simulink model "clik_inverse"  (Simulink 10.2)
settings: Solver=ode1  StartTime=0.0  StopTime=4  FixedStep=0.001  RelTol=1e-3
undefined symbols (not defined in the file or in its folder): DiscIntNeverNeededParam, q0, Tc
settings Model: Creator=Xp  LastModifiedBy=Megha
settings DataIOCC: LimitDataPoints=on
settings OptimizationCC: ExpressionDepthLimit=2147483647  InitFltsAndDblsToZero=on
settings DebuggingCC: SaveWithParameterizedLinksMsg=none  SolverPrmCheckMsg=warning  MultiTaskDSMMsg=warning  MultiTaskCondExecSysMsg=none  StateNameClashWarn=warning
settings SFSimCC: SimUseLocalCustomCode=on
settings RTWCC: RTWUseLocalCustomCode=on
settings ConfigComp: CovExternalEMLEnable=on

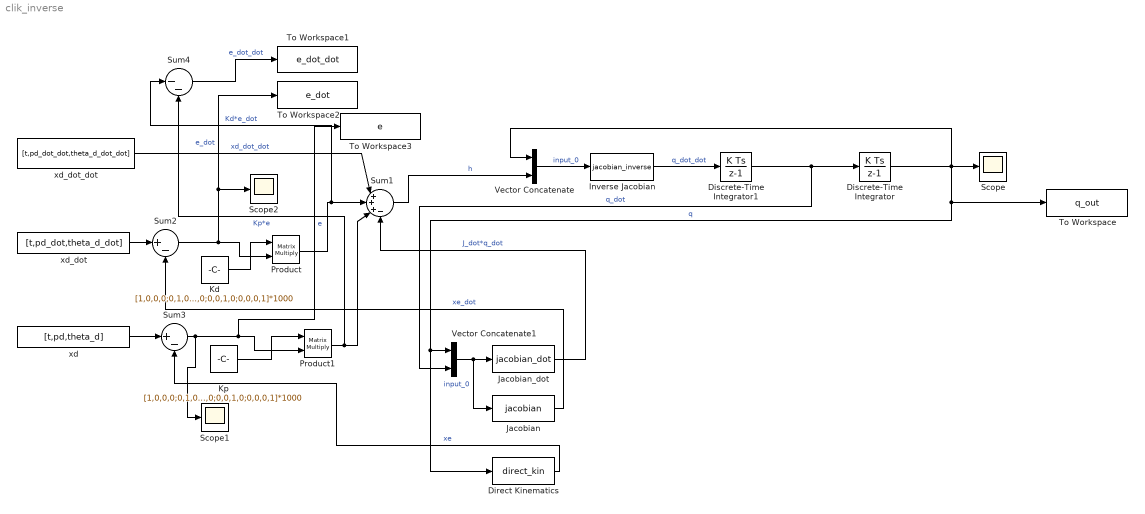
== system clik_inverse ==
  Direct Kinematics : MATLABFcn  MATLABFcn=direct_kin  Output1D=off
  Discrete-Time Integrator : DiscreteIntegrator  InitialCondition=q0  SampleTime=Tc  ICPrevOutput=DiscIntNeverNeededParam  ICPrevScaledInput=DiscIntNeverNeededParam
  Discrete-Time Integrator1 : DiscreteIntegrator  InitialCondition=[0;0;0;0]  SampleTime=Tc  ICPrevOutput=DiscIntNeverNeededParam  ICPrevScaledInput=DiscIntNeverNeededParam
  Inverse Jacobian : MATLABFcn  MATLABFcn=jacobian_inverse  Output1D=off
  Jacobian : MATLABFcn  MATLABFcn=jacobian  Output1D=off
  Jacobian_dot : MATLABFcn  MATLABFcn=jacobian_dot  OutputDimensions=[4,1]  Output1D=off
  Kd : Constant  Value=[1,0,0,0;0,1,0,0;0,0,1,0;0,0,0,1]*1000  VectorParams1D=off
  Kp : Constant  Value=[1,0,0,0;0,1,0,0;0,0,1,0;0,0,0,1]*1000  VectorParams1D=off
  Product : Product  Multiplication=Matrix(*)
  Product1 : Product  Multiplication=Matrix(*)
  Scope : Scope
  Scope1 : Scope
  Scope2 : Scope
  Sum1 : Sum  Inputs=|+++-
  Sum2 : Sum  Inputs=|+-
  Sum3 : Sum  Inputs=|+-
  Sum4 : Sum  Inputs=|--
  To Workspace : ToWorkspace  VariableName=q_out  SampleTime=Tc
  To Workspace1 : ToWorkspace  VariableName=e_dot_dot  SampleTime=Tc
  To Workspace2 : ToWorkspace  VariableName=e_dot  SampleTime=-1
  To Workspace3 : ToWorkspace  VariableName=e  SampleTime=Tc
  Vector Concatenate : Concatenate
  Vector Concatenate1 : Concatenate
  xd : FromWorkspace  VariableName=[t,pd,theta_d]
  xd_dot : FromWorkspace  VariableName=[t,pd_dot,theta_d_dot]
  xd_dot_dot : FromWorkspace  VariableName=[t,pd_dot_dot,theta_d_dot_dot]
  wires:
  Discrete-Time Integrator1/1 -> Vector Concatenate1/2, Discrete-Time Integrator/1  "q_dot"
  Inverse Jacobian/1 -> Discrete-Time Integrator1/1  "q_dot_dot"
  xd_dot_dot/1 -> Sum1/1  "xd_dot_dot"
  Sum1/1 -> Vector Concatenate/2  "h"
  Discrete-Time Integrator/1 -> To Workspace/1, Direct Kinematics/1, Vector Concatenate1/1, Vector Concatenate/1, Scope/1  "q"
  Jacobian/1 -> Sum2/2  "xe_dot"
  Direct Kinematics/1 -> Sum3/2  "xe"
  Jacobian_dot/1 -> Sum1/4  "J_dot*q_dot"
  xd_dot/1 -> Sum2/1
  Sum2/1 -> Product/2, To Workspace2/1, Scope2/1  "e_dot"
  Product/1 -> Sum4/1, Sum1/2  "Kd*e_dot"
  xd/1 -> Sum3/1
  Sum3/1 -> To Workspace3/1, Product1/2, Scope1/1  "e"
  Product1/1 -> Sum4/2, Sum1/3  "Kp*e"
  Vector Concatenate/1 -> Inverse Jacobian/1  "input_0"
  Kd/1 -> Product/1
  Kp/1 -> Product1/1
  Vector Concatenate1/1 -> Jacobian/1, Jacobian_dot/1  "input_0"
  Sum4/1 -> To Workspace1/1  "e_dot_dot"
